simulink model "sudoku"  (R2012b)
settings: Solver=ode45  StartTime=0.0  StopTime=10.0  RelTol=1e-3
libraries: sldvlib x83
(part 4 of 4)

== system sudoku/blocks/block_5 ==
  In1 : Inport
  In2 : Inport  Port=2
  In3 : Inport  Port=3
  In4 : Inport  Port=4
  In5 : Inport  Port=5
  In6 : Inport  Port=6
  In7 : Inport  Port=7
  In8 : Inport  Port=8
  In9 : Inport  Port=9
  Logical Operator : Logic  Inputs=8  AllPortsSameDT=off  OutDataTypeStr=boolean
  Logical Operator1 : Logic  Inputs=7  AllPortsSameDT=off  OutDataTypeStr=boolean
  Logical Operator2 : Logic  Inputs=6  AllPortsSameDT=off  OutDataTypeStr=boolean
  Logical Operator3 : Logic  Inputs=5  AllPortsSameDT=off  OutDataTypeStr=boolean
  Logical Operator4 : Logic  Inputs=4  AllPortsSameDT=off  OutDataTypeStr=boolean
  Logical Operator5 : Logic  Inputs=3  AllPortsSameDT=off  OutDataTypeStr=boolean
  Logical Operator6 : Logic  AllPortsSameDT=off  OutDataTypeStr=boolean
  Logical Operator7 : Logic  Inputs=8  AllPortsSameDT=off  OutDataTypeStr=boolean
  diff{1..36} (36 alike) : RelationalOperator  Operator=~=  OutDataTypeStr=boolean
  Out1 : Outport
  wires:
  In2/1 -> diff1/2, diff15/1, diff14/1, diff13/1, diff12/1, diff11/1, diff10/1, diff9/1
  In1/1 -> diff8/1, diff7/1, diff6/1, diff5/1, diff4/1, diff3/1, diff2/1, diff1/1
  In5/1 -> diff30/1, diff29/1, diff28/1, diff27/1, diff22/2, diff17/2, diff11/2, diff4/2
  In6/1 -> diff33/1, diff32/1, diff31/1, diff27/2, diff23/2, diff18/2, diff12/2, diff5/2
  In7/1 -> diff19/2, diff35/1, diff34/1, diff31/2, diff28/2, diff24/2, diff13/2, diff6/2
  diff1/1 -> Logical Operator/1
  In3/1 -> diff2/2, diff21/1, diff20/1, diff19/1, diff18/1, diff17/1, diff16/1, diff9/2
  In4/1 -> diff26/1, diff25/1, diff24/1, diff23/1, diff22/1, diff16/2, diff10/2, diff3/2
  diff8/1 -> Logical Operator/8
  diff26/1 -> Logical Operator3/5
  diff36/1 -> Logical Operator7/1
  Logical Operator1/1 -> Logical Operator7/7
  diff10/1 -> Logical Operator1/2
  diff18/1 -> Logical Operator2/3
  diff17/1 -> Logical Operator2/2
  diff31/1 -> Logical Operator5/1
  Logical Operator5/1 -> Logical Operator7/3
  diff34/1 -> Logical Operator6/1
  diff16/1 -> Logical Operator2/1
  diff33/1 -> Logical Operator5/3
  diff22/1 -> Logical Operator3/1
  diff35/1 -> Logical Operator6/2
  diff27/1 -> Logical Operator4/1
  Logical Operator/1 -> Logical Operator7/8
  diff25/1 -> Logical Operator3/4
  diff3/1 -> Logical Operator/3
  diff2/1 -> Logical Operator/2
  diff7/1 -> Logical Operator/7
  diff5/1 -> Logical Operator/5
  diff4/1 -> Logical Operator/4
  diff30/1 -> Logical Operator4/4
  Logical Operator7/1 -> Out1/1
  Logical Operator3/1 -> Logical Operator7/5
  Logical Operator6/1 -> Logical Operator7/2
  diff14/1 -> Logical Operator1/6
  Logical Operator2/1 -> Logical Operator7/6
  diff15/1 -> Logical Operator1/7
  diff32/1 -> Logical Operator5/2
  diff21/1 -> Logical Operator2/6
  Logical Operator4/1 -> Logical Operator7/4
  diff19/1 -> Logical Operator2/4
  diff20/1 -> Logical Operator2/5
  diff28/1 -> Logical Operator4/2
  In8/1 -> diff29/2, diff36/1, diff34/2, diff32/2, diff25/2, diff20/2, diff14/2, diff7/2
  diff29/1 -> Logical Operator4/3
  diff6/1 -> Logical Operator/6
  diff9/1 -> Logical Operator1/1
  diff23/1 -> Logical Operator3/2
  diff13/1 -> Logical Operator1/5
  diff24/1 -> Logical Operator3/3
  diff11/1 -> Logical Operator1/3
  diff12/1 -> Logical Operator1/4
  In9/1 -> diff35/2, diff36/2, diff33/2, diff30/2, diff26/2, diff21/2, diff15/2, diff8/2

== system sudoku/blocks/block_6 ==
  In1 : Inport
  In2 : Inport  Port=2
  In3 : Inport  Port=3
  In4 : Inport  Port=4
  In5 : Inport  Port=5
  In6 : Inport  Port=6
  In7 : Inport  Port=7
  In8 : Inport  Port=8
  In9 : Inport  Port=9
  Logical Operator : Logic  Inputs=8  AllPortsSameDT=off  OutDataTypeStr=boolean
  Logical Operator1 : Logic  Inputs=7  AllPortsSameDT=off  OutDataTypeStr=boolean
  Logical Operator2 : Logic  Inputs=6  AllPortsSameDT=off  OutDataTypeStr=boolean
  Logical Operator3 : Logic  Inputs=5  AllPortsSameDT=off  OutDataTypeStr=boolean
  Logical Operator4 : Logic  Inputs=4  AllPortsSameDT=off  OutDataTypeStr=boolean
  Logical Operator5 : Logic  Inputs=3  AllPortsSameDT=off  OutDataTypeStr=boolean
  Logical Operator6 : Logic  AllPortsSameDT=off  OutDataTypeStr=boolean
  Logical Operator7 : Logic  Inputs=8  AllPortsSameDT=off  OutDataTypeStr=boolean
  diff{1..36} (36 alike) : RelationalOperator  Operator=~=  OutDataTypeStr=boolean
  Out1 : Outport
  wires:
  In2/1 -> diff1/2, diff15/1, diff14/1, diff13/1, diff12/1, diff11/1, diff10/1, diff9/1
  In1/1 -> diff8/1, diff7/1, diff6/1, diff5/1, diff4/1, diff3/1, diff2/1, diff1/1
  In5/1 -> diff30/1, diff29/1, diff28/1, diff27/1, diff22/2, diff17/2, diff11/2, diff4/2
  In6/1 -> diff33/1, diff32/1, diff31/1, diff27/2, diff23/2, diff18/2, diff12/2, diff5/2
  In7/1 -> diff19/2, diff35/1, diff34/1, diff31/2, diff28/2, diff24/2, diff13/2, diff6/2
  diff1/1 -> Logical Operator/1
  In3/1 -> diff2/2, diff21/1, diff20/1, diff19/1, diff18/1, diff17/1, diff16/1, diff9/2
  In4/1 -> diff26/1, diff25/1, diff24/1, diff23/1, diff22/1, diff16/2, diff10/2, diff3/2
  diff8/1 -> Logical Operator/8
  diff26/1 -> Logical Operator3/5
  diff36/1 -> Logical Operator7/1
  Logical Operator1/1 -> Logical Operator7/7
  diff10/1 -> Logical Operator1/2
  diff18/1 -> Logical Operator2/3
  diff17/1 -> Logical Operator2/2
  diff31/1 -> Logical Operator5/1
  Logical Operator5/1 -> Logical Operator7/3
  diff34/1 -> Logical Operator6/1
  diff16/1 -> Logical Operator2/1
  diff33/1 -> Logical Operator5/3
  diff22/1 -> Logical Operator3/1
  diff35/1 -> Logical Operator6/2
  diff27/1 -> Logical Operator4/1
  Logical Operator/1 -> Logical Operator7/8
  diff25/1 -> Logical Operator3/4
  diff3/1 -> Logical Operator/3
  diff2/1 -> Logical Operator/2
  diff7/1 -> Logical Operator/7
  diff5/1 -> Logical Operator/5
  diff4/1 -> Logical Operator/4
  diff30/1 -> Logical Operator4/4
  Logical Operator7/1 -> Out1/1
  Logical Operator3/1 -> Logical Operator7/5
  Logical Operator6/1 -> Logical Operator7/2
  diff14/1 -> Logical Operator1/6
  Logical Operator2/1 -> Logical Operator7/6
  diff15/1 -> Logical Operator1/7
  diff32/1 -> Logical Operator5/2
  diff21/1 -> Logical Operator2/6
  Logical Operator4/1 -> Logical Operator7/4
  diff19/1 -> Logical Operator2/4
  diff20/1 -> Logical Operator2/5
  diff28/1 -> Logical Operator4/2
  In8/1 -> diff29/2, diff36/1, diff34/2, diff32/2, diff25/2, diff20/2, diff14/2, diff7/2
  diff29/1 -> Logical Operator4/3
  diff6/1 -> Logical Operator/6
  diff9/1 -> Logical Operator1/1
  diff23/1 -> Logical Operator3/2
  diff13/1 -> Logical Operator1/5
  diff24/1 -> Logical Operator3/3
  diff11/1 -> Logical Operator1/3
  diff12/1 -> Logical Operator1/4
  In9/1 -> diff35/2, diff36/2, diff33/2, diff30/2, diff26/2, diff21/2, diff15/2, diff8/2

== system sudoku/blocks/block_7 ==
  In1 : Inport
  In2 : Inport  Port=2
  In3 : Inport  Port=3
  In4 : Inport  Port=4
  In5 : Inport  Port=5
  In6 : Inport  Port=6
  In7 : Inport  Port=7
  In8 : Inport  Port=8
  In9 : Inport  Port=9
  Logical Operator : Logic  Inputs=8  AllPortsSameDT=off  OutDataTypeStr=boolean
  Logical Operator1 : Logic  Inputs=7  AllPortsSameDT=off  OutDataTypeStr=boolean
  Logical Operator2 : Logic  Inputs=6  AllPortsSameDT=off  OutDataTypeStr=boolean
  Logical Operator3 : Logic  Inputs=5  AllPortsSameDT=off  OutDataTypeStr=boolean
  Logical Operator4 : Logic  Inputs=4  AllPortsSameDT=off  OutDataTypeStr=boolean
  Logical Operator5 : Logic  Inputs=3  AllPortsSameDT=off  OutDataTypeStr=boolean
  Logical Operator6 : Logic  AllPortsSameDT=off  OutDataTypeStr=boolean
  Logical Operator7 : Logic  Inputs=8  AllPortsSameDT=off  OutDataTypeStr=boolean
  diff{1..36} (36 alike) : RelationalOperator  Operator=~=  OutDataTypeStr=boolean
  Out1 : Outport
  wires:
  In2/1 -> diff1/2, diff15/1, diff14/1, diff13/1, diff12/1, diff11/1, diff10/1, diff9/1
  In1/1 -> diff8/1, diff7/1, diff6/1, diff5/1, diff4/1, diff3/1, diff2/1, diff1/1
  In5/1 -> diff30/1, diff29/1, diff28/1, diff27/1, diff22/2, diff17/2, diff11/2, diff4/2
  In6/1 -> diff33/1, diff32/1, diff31/1, diff27/2, diff23/2, diff18/2, diff12/2, diff5/2
  In7/1 -> diff19/2, diff35/1, diff34/1, diff31/2, diff28/2, diff24/2, diff13/2, diff6/2
  diff1/1 -> Logical Operator/1
  In3/1 -> diff2/2, diff21/1, diff20/1, diff19/1, diff18/1, diff17/1, diff16/1, diff9/2
  In4/1 -> diff26/1, diff25/1, diff24/1, diff23/1, diff22/1, diff16/2, diff10/2, diff3/2
  diff8/1 -> Logical Operator/8
  diff26/1 -> Logical Operator3/5
  diff36/1 -> Logical Operator7/1
  Logical Operator1/1 -> Logical Operator7/7
  diff10/1 -> Logical Operator1/2
  diff18/1 -> Logical Operator2/3
  diff17/1 -> Logical Operator2/2
  diff31/1 -> Logical Operator5/1
  Logical Operator5/1 -> Logical Operator7/3
  diff34/1 -> Logical Operator6/1
  diff16/1 -> Logical Operator2/1
  diff33/1 -> Logical Operator5/3
  diff22/1 -> Logical Operator3/1
  diff35/1 -> Logical Operator6/2
  diff27/1 -> Logical Operator4/1
  Logical Operator/1 -> Logical Operator7/8
  diff25/1 -> Logical Operator3/4
  diff3/1 -> Logical Operator/3
  diff2/1 -> Logical Operator/2
  diff7/1 -> Logical Operator/7
  diff5/1 -> Logical Operator/5
  diff4/1 -> Logical Operator/4
  diff30/1 -> Logical Operator4/4
  Logical Operator7/1 -> Out1/1
  Logical Operator3/1 -> Logical Operator7/5
  Logical Operator6/1 -> Logical Operator7/2
  diff14/1 -> Logical Operator1/6
  Logical Operator2/1 -> Logical Operator7/6
  diff15/1 -> Logical Operator1/7
  diff32/1 -> Logical Operator5/2
  diff21/1 -> Logical Operator2/6
  Logical Operator4/1 -> Logical Operator7/4
  diff19/1 -> Logical Operator2/4
  diff20/1 -> Logical Operator2/5
  diff28/1 -> Logical Operator4/2
  In8/1 -> diff29/2, diff36/1, diff34/2, diff32/2, diff25/2, diff20/2, diff14/2, diff7/2
  diff29/1 -> Logical Operator4/3
  diff6/1 -> Logical Operator/6
  diff9/1 -> Logical Operator1/1
  diff23/1 -> Logical Operator3/2
  diff13/1 -> Logical Operator1/5
  diff24/1 -> Logical Operator3/3
  diff11/1 -> Logical Operator1/3
  diff12/1 -> Logical Operator1/4
  In9/1 -> diff35/2, diff36/2, diff33/2, diff30/2, diff26/2, diff21/2, diff15/2, diff8/2

== system sudoku/blocks/block_8 ==
  In1 : Inport
  In2 : Inport  Port=2
  In3 : Inport  Port=3
  In4 : Inport  Port=4
  In5 : Inport  Port=5
  In6 : Inport  Port=6
  In7 : Inport  Port=7
  In8 : Inport  Port=8
  In9 : Inport  Port=9
  Logical Operator : Logic  Inputs=8  AllPortsSameDT=off  OutDataTypeStr=boolean
  Logical Operator1 : Logic  Inputs=7  AllPortsSameDT=off  OutDataTypeStr=boolean
  Logical Operator2 : Logic  Inputs=6  AllPortsSameDT=off  OutDataTypeStr=boolean
  Logical Operator3 : Logic  Inputs=5  AllPortsSameDT=off  OutDataTypeStr=boolean
  Logical Operator4 : Logic  Inputs=4  AllPortsSameDT=off  OutDataTypeStr=boolean
  Logical Operator5 : Logic  Inputs=3  AllPortsSameDT=off  OutDataTypeStr=boolean
  Logical Operator6 : Logic  AllPortsSameDT=off  OutDataTypeStr=boolean
  Logical Operator7 : Logic  Inputs=8  AllPortsSameDT=off  OutDataTypeStr=boolean
  diff{1..36} (36 alike) : RelationalOperator  Operator=~=  OutDataTypeStr=boolean
  Out1 : Outport
  wires:
  In2/1 -> diff1/2, diff15/1, diff14/1, diff13/1, diff12/1, diff11/1, diff10/1, diff9/1
  In1/1 -> diff8/1, diff7/1, diff6/1, diff5/1, diff4/1, diff3/1, diff2/1, diff1/1
  In5/1 -> diff30/1, diff29/1, diff28/1, diff27/1, diff22/2, diff17/2, diff11/2, diff4/2
  In6/1 -> diff33/1, diff32/1, diff31/1, diff27/2, diff23/2, diff18/2, diff12/2, diff5/2
  In7/1 -> diff19/2, diff35/1, diff34/1, diff31/2, diff28/2, diff24/2, diff13/2, diff6/2
  diff1/1 -> Logical Operator/1
  In3/1 -> diff2/2, diff21/1, diff20/1, diff19/1, diff18/1, diff17/1, diff16/1, diff9/2
  In4/1 -> diff26/1, diff25/1, diff24/1, diff23/1, diff22/1, diff16/2, diff10/2, diff3/2
  diff8/1 -> Logical Operator/8
  diff26/1 -> Logical Operator3/5
  diff36/1 -> Logical Operator7/1
  Logical Operator1/1 -> Logical Operator7/7
  diff10/1 -> Logical Operator1/2
  diff18/1 -> Logical Operator2/3
  diff17/1 -> Logical Operator2/2
  diff31/1 -> Logical Operator5/1
  Logical Operator5/1 -> Logical Operator7/3
  diff34/1 -> Logical Operator6/1
  diff16/1 -> Logical Operator2/1
  diff33/1 -> Logical Operator5/3
  diff22/1 -> Logical Operator3/1
  diff35/1 -> Logical Operator6/2
  diff27/1 -> Logical Operator4/1
  Logical Operator/1 -> Logical Operator7/8
  diff25/1 -> Logical Operator3/4
  diff3/1 -> Logical Operator/3
  diff2/1 -> Logical Operator/2
  diff7/1 -> Logical Operator/7
  diff5/1 -> Logical Operator/5
  diff4/1 -> Logical Operator/4
  diff30/1 -> Logical Operator4/4
  Logical Operator7/1 -> Out1/1
  Logical Operator3/1 -> Logical Operator7/5
  Logical Operator6/1 -> Logical Operator7/2
  diff14/1 -> Logical Operator1/6
  Logical Operator2/1 -> Logical Operator7/6
  diff15/1 -> Logical Operator1/7
  diff32/1 -> Logical Operator5/2
  diff21/1 -> Logical Operator2/6
  Logical Operator4/1 -> Logical Operator7/4
  diff19/1 -> Logical Operator2/4
  diff20/1 -> Logical Operator2/5
  diff28/1 -> Logical Operator4/2
  In8/1 -> diff29/2, diff36/1, diff34/2, diff32/2, diff25/2, diff20/2, diff14/2, diff7/2
  diff29/1 -> Logical Operator4/3
  diff6/1 -> Logical Operator/6
  diff9/1 -> Logical Operator1/1
  diff23/1 -> Logical Operator3/2
  diff13/1 -> Logical Operator1/5
  diff24/1 -> Logical Operator3/3
  diff11/1 -> Logical Operator1/3
  diff12/1 -> Logical Operator1/4
  In9/1 -> diff35/2, diff36/2, diff33/2, diff30/2, diff26/2, diff21/2, diff15/2, diff8/2

== system sudoku/blocks/block_9 ==
  In1 : Inport
  In2 : Inport  Port=2
  In3 : Inport  Port=3
  In4 : Inport  Port=4
  In5 : Inport  Port=5
  In6 : Inport  Port=6
  In7 : Inport  Port=7
  In8 : Inport  Port=8
  In9 : Inport  Port=9
  Logical Operator : Logic  Inputs=8  AllPortsSameDT=off  OutDataTypeStr=boolean
  Logical Operator1 : Logic  Inputs=7  AllPortsSameDT=off  OutDataTypeStr=boolean
  Logical Operator2 : Logic  Inputs=6  AllPortsSameDT=off  OutDataTypeStr=boolean
  Logical Operator3 : Logic  Inputs=5  AllPortsSameDT=off  OutDataTypeStr=boolean
  Logical Operator4 : Logic  Inputs=4  AllPortsSameDT=off  OutDataTypeStr=boolean
  Logical Operator5 : Logic  Inputs=3  AllPortsSameDT=off  OutDataTypeStr=boolean
  Logical Operator6 : Logic  AllPortsSameDT=off  OutDataTypeStr=boolean
  Logical Operator7 : Logic  Inputs=8  AllPortsSameDT=off  OutDataTypeStr=boolean
  diff{1..36} (36 alike) : RelationalOperator  Operator=~=  OutDataTypeStr=boolean
  Out1 : Outport
  wires:
  In2/1 -> diff1/2, diff15/1, diff14/1, diff13/1, diff12/1, diff11/1, diff10/1, diff9/1
  In1/1 -> diff8/1, diff7/1, diff6/1, diff5/1, diff4/1, diff3/1, diff2/1, diff1/1
  In5/1 -> diff30/1, diff29/1, diff28/1, diff27/1, diff22/2, diff17/2, diff11/2, diff4/2
  In6/1 -> diff33/1, diff32/1, diff31/1, diff27/2, diff23/2, diff18/2, diff12/2, diff5/2
  In7/1 -> diff19/2, diff35/1, diff34/1, diff31/2, diff28/2, diff24/2, diff13/2, diff6/2
  diff1/1 -> Logical Operator/1
  In3/1 -> diff2/2, diff21/1, diff20/1, diff19/1, diff18/1, diff17/1, diff16/1, diff9/2
  In4/1 -> diff26/1, diff25/1, diff24/1, diff23/1, diff22/1, diff16/2, diff10/2, diff3/2
  diff8/1 -> Logical Operator/8
  diff26/1 -> Logical Operator3/5
  diff36/1 -> Logical Operator7/1
  Logical Operator1/1 -> Logical Operator7/7
  diff10/1 -> Logical Operator1/2
  diff18/1 -> Logical Operator2/3
  diff17/1 -> Logical Operator2/2
  diff31/1 -> Logical Operator5/1
  Logical Operator5/1 -> Logical Operator7/3
  diff34/1 -> Logical Operator6/1
  diff16/1 -> Logical Operator2/1
  diff33/1 -> Logical Operator5/3
  diff22/1 -> Logical Operator3/1
  diff35/1 -> Logical Operator6/2
  diff27/1 -> Logical Operator4/1
  Logical Operator/1 -> Logical Operator7/8
  diff25/1 -> Logical Operator3/4
  diff3/1 -> Logical Operator/3
  diff2/1 -> Logical Operator/2
  diff7/1 -> Logical Operator/7
  diff5/1 -> Logical Operator/5
  diff4/1 -> Logical Operator/4
  diff30/1 -> Logical Operator4/4
  Logical Operator7/1 -> Out1/1
  Logical Operator3/1 -> Logical Operator7/5
  Logical Operator6/1 -> Logical Operator7/2
  diff14/1 -> Logical Operator1/6
  Logical Operator2/1 -> Logical Operator7/6
  diff15/1 -> Logical Operator1/7
  diff32/1 -> Logical Operator5/2
  diff21/1 -> Logical Operator2/6
  Logical Operator4/1 -> Logical Operator7/4
  diff19/1 -> Logical Operator2/4
  diff20/1 -> Logical Operator2/5
  diff28/1 -> Logical Operator4/2
  In8/1 -> diff29/2, diff36/1, diff34/2, diff32/2, diff25/2, diff20/2, diff14/2, diff7/2
  diff29/1 -> Logical Operator4/3
  diff6/1 -> Logical Operator/6
  diff9/1 -> Logical Operator1/1
  diff23/1 -> Logical Operator3/2
  diff13/1 -> Logical Operator1/5
  diff24/1 -> Logical Operator3/3
  diff11/1 -> Logical Operator1/3
  diff12/1 -> Logical Operator1/4
  In9/1 -> diff35/2, diff36/2, diff33/2, diff30/2, diff26/2, diff21/2, diff15/2, diff8/2

== system sudoku/columns/col_1 ==
  In1 : Inport
  In2 : Inport  Port=2
  In3 : Inport  Port=3
  In4 : Inport  Port=4
  In5 : Inport  Port=5
  In6 : Inport  Port=6
  In7 : Inport  Port=7
  In8 : Inport  Port=8
  In9 : Inport  Port=9
  Logical Operator : Logic  Inputs=8  AllPortsSameDT=off  OutDataTypeStr=boolean
  Logical Operator1 : Logic  Inputs=7  AllPortsSameDT=off  OutDataTypeStr=boolean
  Logical Operator2 : Logic  Inputs=6  AllPortsSameDT=off  OutDataTypeStr=boolean
  Logical Operator3 : Logic  Inputs=5  AllPortsSameDT=off  OutDataTypeStr=boolean
  Logical Operator4 : Logic  Inputs=4  AllPortsSameDT=off  OutDataTypeStr=boolean
  Logical Operator5 : Logic  Inputs=3  AllPortsSameDT=off  OutDataTypeStr=boolean
  Logical Operator6 : Logic  AllPortsSameDT=off  OutDataTypeStr=boolean
  Logical Operator7 : Logic  Inputs=8  AllPortsSameDT=off  OutDataTypeStr=boolean
  diff{1..36} (36 alike) : RelationalOperator  Operator=~=  OutDataTypeStr=boolean
  Out1 : Outport
  wires:
  In2/1 -> diff1/2, diff15/1, diff14/1, diff13/1, diff12/1, diff11/1, diff10/1, diff9/1
  In1/1 -> diff8/1, diff7/1, diff6/1, diff5/1, diff4/1, diff3/1, diff2/1, diff1/1
  In5/1 -> diff30/1, diff29/1, diff28/1, diff27/1, diff22/2, diff17/2, diff11/2, diff4/2
  In6/1 -> diff33/1, diff32/1, diff31/1, diff27/2, diff23/2, diff18/2, diff12/2, diff5/2
  In7/1 -> diff19/2, diff35/1, diff34/1, diff31/2, diff28/2, diff24/2, diff13/2, diff6/2
  diff1/1 -> Logical Operator/1
  In3/1 -> diff2/2, diff21/1, diff20/1, diff19/1, diff18/1, diff17/1, diff16/1, diff9/2
  In4/1 -> diff26/1, diff25/1, diff24/1, diff23/1, diff22/1, diff16/2, diff10/2, diff3/2
  diff8/1 -> Logical Operator/8
  diff26/1 -> Logical Operator3/5
  diff36/1 -> Logical Operator7/1
  Logical Operator1/1 -> Logical Operator7/7
  diff10/1 -> Logical Operator1/2
  diff18/1 -> Logical Operator2/3
  diff17/1 -> Logical Operator2/2
  diff31/1 -> Logical Operator5/1
  Logical Operator5/1 -> Logical Operator7/3
  diff34/1 -> Logical Operator6/1
  diff16/1 -> Logical Operator2/1
  diff33/1 -> Logical Operator5/3
  diff22/1 -> Logical Operator3/1
  diff35/1 -> Logical Operator6/2
  diff27/1 -> Logical Operator4/1
  Logical Operator/1 -> Logical Operator7/8
  diff25/1 -> Logical Operator3/4
  diff3/1 -> Logical Operator/3
  diff2/1 -> Logical Operator/2
  diff7/1 -> Logical Operator/7
  diff5/1 -> Logical Operator/5
  diff4/1 -> Logical Operator/4
  diff30/1 -> Logical Operator4/4
  Logical Operator7/1 -> Out1/1
  Logical Operator3/1 -> Logical Operator7/5
  Logical Operator6/1 -> Logical Operator7/2
  diff14/1 -> Logical Operator1/6
  Logical Operator2/1 -> Logical Operator7/6
  diff15/1 -> Logical Operator1/7
  diff32/1 -> Logical Operator5/2
  diff21/1 -> Logical Operator2/6
  Logical Operator4/1 -> Logical Operator7/4
  diff19/1 -> Logical Operator2/4
  diff20/1 -> Logical Operator2/5
  diff28/1 -> Logical Operator4/2
  In8/1 -> diff29/2, diff36/1, diff34/2, diff32/2, diff25/2, diff20/2, diff14/2, diff7/2
  diff29/1 -> Logical Operator4/3
  diff6/1 -> Logical Operator/6
  diff9/1 -> Logical Operator1/1
  diff23/1 -> Logical Operator3/2
  diff13/1 -> Logical Operator1/5
  diff24/1 -> Logical Operator3/3
  diff11/1 -> Logical Operator1/3
  diff12/1 -> Logical Operator1/4
  In9/1 -> diff35/2, diff36/2, diff33/2, diff30/2, diff26/2, diff21/2, diff15/2, diff8/2

== system sudoku/columns/col_2 ==
  In1 : Inport
  In2 : Inport  Port=2
  In3 : Inport  Port=3
  In4 : Inport  Port=4
  In5 : Inport  Port=5
  In6 : Inport  Port=6
  In7 : Inport  Port=7
  In8 : Inport  Port=8
  In9 : Inport  Port=9
  Logical Operator : Logic  Inputs=8  AllPortsSameDT=off  OutDataTypeStr=boolean
  Logical Operator1 : Logic  Inputs=7  AllPortsSameDT=off  OutDataTypeStr=boolean
  Logical Operator2 : Logic  Inputs=6  AllPortsSameDT=off  OutDataTypeStr=boolean
  Logical Operator3 : Logic  Inputs=5  AllPortsSameDT=off  OutDataTypeStr=boolean
  Logical Operator4 : Logic  Inputs=4  AllPortsSameDT=off  OutDataTypeStr=boolean
  Logical Operator5 : Logic  Inputs=3  AllPortsSameDT=off  OutDataTypeStr=boolean
  Logical Operator6 : Logic  AllPortsSameDT=off  OutDataTypeStr=boolean
  Logical Operator7 : Logic  Inputs=8  AllPortsSameDT=off  OutDataTypeStr=boolean
  diff{1..36} (36 alike) : RelationalOperator  Operator=~=  OutDataTypeStr=boolean
  Out1 : Outport
  wires:
  In2/1 -> diff1/2, diff15/1, diff14/1, diff13/1, diff12/1, diff11/1, diff10/1, diff9/1
  In1/1 -> diff8/1, diff7/1, diff6/1, diff5/1, diff4/1, diff3/1, diff2/1, diff1/1
  In5/1 -> diff30/1, diff29/1, diff28/1, diff27/1, diff22/2, diff17/2, diff11/2, diff4/2
  In6/1 -> diff33/1, diff32/1, diff31/1, diff27/2, diff23/2, diff18/2, diff12/2, diff5/2
  In7/1 -> diff19/2, diff35/1, diff34/1, diff31/2, diff28/2, diff24/2, diff13/2, diff6/2
  diff1/1 -> Logical Operator/1
  In3/1 -> diff2/2, diff21/1, diff20/1, diff19/1, diff18/1, diff17/1, diff16/1, diff9/2
  In4/1 -> diff26/1, diff25/1, diff24/1, diff23/1, diff22/1, diff16/2, diff10/2, diff3/2
  diff8/1 -> Logical Operator/8
  diff26/1 -> Logical Operator3/5
  diff36/1 -> Logical Operator7/1
  Logical Operator1/1 -> Logical Operator7/7
  diff10/1 -> Logical Operator1/2
  diff18/1 -> Logical Operator2/3
  diff17/1 -> Logical Operator2/2
  diff31/1 -> Logical Operator5/1
  Logical Operator5/1 -> Logical Operator7/3
  diff34/1 -> Logical Operator6/1
  diff16/1 -> Logical Operator2/1
  diff33/1 -> Logical Operator5/3
  diff22/1 -> Logical Operator3/1
  diff35/1 -> Logical Operator6/2
  diff27/1 -> Logical Operator4/1
  Logical Operator/1 -> Logical Operator7/8
  diff25/1 -> Logical Operator3/4
  diff3/1 -> Logical Operator/3
  diff2/1 -> Logical Operator/2
  diff7/1 -> Logical Operator/7
  diff5/1 -> Logical Operator/5
  diff4/1 -> Logical Operator/4
  diff30/1 -> Logical Operator4/4
  Logical Operator7/1 -> Out1/1
  Logical Operator3/1 -> Logical Operator7/5
  Logical Operator6/1 -> Logical Operator7/2
  diff14/1 -> Logical Operator1/6
  Logical Operator2/1 -> Logical Operator7/6
  diff15/1 -> Logical Operator1/7
  diff32/1 -> Logical Operator5/2
  diff21/1 -> Logical Operator2/6
  Logical Operator4/1 -> Logical Operator7/4
  diff19/1 -> Logical Operator2/4
  diff20/1 -> Logical Operator2/5
  diff28/1 -> Logical Operator4/2
  In8/1 -> diff29/2, diff36/1, diff34/2, diff32/2, diff25/2, diff20/2, diff14/2, diff7/2
  diff29/1 -> Logical Operator4/3
  diff6/1 -> Logical Operator/6
  diff9/1 -> Logical Operator1/1
  diff23/1 -> Logical Operator3/2
  diff13/1 -> Logical Operator1/5
  diff24/1 -> Logical Operator3/3
  diff11/1 -> Logical Operator1/3
  diff12/1 -> Logical Operator1/4
  In9/1 -> diff35/2, diff36/2, diff33/2, diff30/2, diff26/2, diff21/2, diff15/2, diff8/2

== system sudoku/columns/col_3 ==
  In1 : Inport
  In2 : Inport  Port=2
  In3 : Inport  Port=3
  In4 : Inport  Port=4
  In5 : Inport  Port=5
  In6 : Inport  Port=6
  In7 : Inport  Port=7
  In8 : Inport  Port=8
  In9 : Inport  Port=9
  Logical Operator : Logic  Inputs=8  AllPortsSameDT=off  OutDataTypeStr=boolean
  Logical Operator1 : Logic  Inputs=7  AllPortsSameDT=off  OutDataTypeStr=boolean
  Logical Operator2 : Logic  Inputs=6  AllPortsSameDT=off  OutDataTypeStr=boolean
  Logical Operator3 : Logic  Inputs=5  AllPortsSameDT=off  OutDataTypeStr=boolean
  Logical Operator4 : Logic  Inputs=4  AllPortsSameDT=off  OutDataTypeStr=boolean
  Logical Operator5 : Logic  Inputs=3  AllPortsSameDT=off  OutDataTypeStr=boolean
  Logical Operator6 : Logic  AllPortsSameDT=off  OutDataTypeStr=boolean
  Logical Operator7 : Logic  Inputs=8  AllPortsSameDT=off  OutDataTypeStr=boolean
  diff{1..36} (36 alike) : RelationalOperator  Operator=~=  OutDataTypeStr=boolean
  Out1 : Outport
  wires:
  In2/1 -> diff1/2, diff15/1, diff14/1, diff13/1, diff12/1, diff11/1, diff10/1, diff9/1
  In1/1 -> diff8/1, diff7/1, diff6/1, diff5/1, diff4/1, diff3/1, diff2/1, diff1/1
  In5/1 -> diff30/1, diff29/1, diff28/1, diff27/1, diff22/2, diff17/2, diff11/2, diff4/2
  In6/1 -> diff33/1, diff32/1, diff31/1, diff27/2, diff23/2, diff18/2, diff12/2, diff5/2
  In7/1 -> diff19/2, diff35/1, diff34/1, diff31/2, diff28/2, diff24/2, diff13/2, diff6/2
  diff1/1 -> Logical Operator/1
  In3/1 -> diff2/2, diff21/1, diff20/1, diff19/1, diff18/1, diff17/1, diff16/1, diff9/2
  In4/1 -> diff26/1, diff25/1, diff24/1, diff23/1, diff22/1, diff16/2, diff10/2, diff3/2
  diff8/1 -> Logical Operator/8
  diff26/1 -> Logical Operator3/5
  diff36/1 -> Logical Operator7/1
  Logical Operator1/1 -> Logical Operator7/7
  diff10/1 -> Logical Operator1/2
  diff18/1 -> Logical Operator2/3
  diff17/1 -> Logical Operator2/2
  diff31/1 -> Logical Operator5/1
  Logical Operator5/1 -> Logical Operator7/3
  diff34/1 -> Logical Operator6/1
  diff16/1 -> Logical Operator2/1
  diff33/1 -> Logical Operator5/3
  diff22/1 -> Logical Operator3/1
  diff35/1 -> Logical Operator6/2
  diff27/1 -> Logical Operator4/1
  Logical Operator/1 -> Logical Operator7/8
  diff25/1 -> Logical Operator3/4
  diff3/1 -> Logical Operator/3
  diff2/1 -> Logical Operator/2
  diff7/1 -> Logical Operator/7
  diff5/1 -> Logical Operator/5
  diff4/1 -> Logical Operator/4
  diff30/1 -> Logical Operator4/4
  Logical Operator7/1 -> Out1/1
  Logical Operator3/1 -> Logical Operator7/5
  Logical Operator6/1 -> Logical Operator7/2
  diff14/1 -> Logical Operator1/6
  Logical Operator2/1 -> Logical Operator7/6
  diff15/1 -> Logical Operator1/7
  diff32/1 -> Logical Operator5/2
  diff21/1 -> Logical Operator2/6
  Logical Operator4/1 -> Logical Operator7/4
  diff19/1 -> Logical Operator2/4
  diff20/1 -> Logical Operator2/5
  diff28/1 -> Logical Operator4/2
  In8/1 -> diff29/2, diff36/1, diff34/2, diff32/2, diff25/2, diff20/2, diff14/2, diff7/2
  diff29/1 -> Logical Operator4/3
  diff6/1 -> Logical Operator/6
  diff9/1 -> Logical Operator1/1
  diff23/1 -> Logical Operator3/2
  diff13/1 -> Logical Operator1/5
  diff24/1 -> Logical Operator3/3
  diff11/1 -> Logical Operator1/3
  diff12/1 -> Logical Operator1/4
  In9/1 -> diff35/2, diff36/2, diff33/2, diff30/2, diff26/2, diff21/2, diff15/2, diff8/2

== system sudoku/columns/col_4 ==
  In1 : Inport
  In2 : Inport  Port=2
  In3 : Inport  Port=3
  In4 : Inport  Port=4
  In5 : Inport  Port=5
  In6 : Inport  Port=6
  In7 : Inport  Port=7
  In8 : Inport  Port=8
  In9 : Inport  Port=9
  Logical Operator : Logic  Inputs=8  AllPortsSameDT=off  OutDataTypeStr=boolean
  Logical Operator1 : Logic  Inputs=7  AllPortsSameDT=off  OutDataTypeStr=boolean
  Logical Operator2 : Logic  Inputs=6  AllPortsSameDT=off  OutDataTypeStr=boolean
  Logical Operator3 : Logic  Inputs=5  AllPortsSameDT=off  OutDataTypeStr=boolean
  Logical Operator4 : Logic  Inputs=4  AllPortsSameDT=off  OutDataTypeStr=boolean
  Logical Operator5 : Logic  Inputs=3  AllPortsSameDT=off  OutDataTypeStr=boolean
  Logical Operator6 : Logic  AllPortsSameDT=off  OutDataTypeStr=boolean
  Logical Operator7 : Logic  Inputs=8  AllPortsSameDT=off  OutDataTypeStr=boolean
  diff{1..36} (36 alike) : RelationalOperator  Operator=~=  OutDataTypeStr=boolean
  Out1 : Outport
  wires:
  In2/1 -> diff1/2, diff15/1, diff14/1, diff13/1, diff12/1, diff11/1, diff10/1, diff9/1
  In1/1 -> diff8/1, diff7/1, diff6/1, diff5/1, diff4/1, diff3/1, diff2/1, diff1/1
  In5/1 -> diff30/1, diff29/1, diff28/1, diff27/1, diff22/2, diff17/2, diff11/2, diff4/2
  In6/1 -> diff33/1, diff32/1, diff31/1, diff27/2, diff23/2, diff18/2, diff12/2, diff5/2
  In7/1 -> diff19/2, diff35/1, diff34/1, diff31/2, diff28/2, diff24/2, diff13/2, diff6/2
  diff1/1 -> Logical Operator/1
  In3/1 -> diff2/2, diff21/1, diff20/1, diff19/1, diff18/1, diff17/1, diff16/1, diff9/2
  In4/1 -> diff26/1, diff25/1, diff24/1, diff23/1, diff22/1, diff16/2, diff10/2, diff3/2
  diff8/1 -> Logical Operator/8
  diff26/1 -> Logical Operator3/5
  diff36/1 -> Logical Operator7/1
  Logical Operator1/1 -> Logical Operator7/7
  diff10/1 -> Logical Operator1/2
  diff18/1 -> Logical Operator2/3
  diff17/1 -> Logical Operator2/2
  diff31/1 -> Logical Operator5/1
  Logical Operator5/1 -> Logical Operator7/3
  diff34/1 -> Logical Operator6/1
  diff16/1 -> Logical Operator2/1
  diff33/1 -> Logical Operator5/3
  diff22/1 -> Logical Operator3/1
  diff35/1 -> Logical Operator6/2
  diff27/1 -> Logical Operator4/1
  Logical Operator/1 -> Logical Operator7/8
  diff25/1 -> Logical Operator3/4
  diff3/1 -> Logical Operator/3
  diff2/1 -> Logical Operator/2
  diff7/1 -> Logical Operator/7
  diff5/1 -> Logical Operator/5
  diff4/1 -> Logical Operator/4
  diff30/1 -> Logical Operator4/4
  Logical Operator7/1 -> Out1/1
  Logical Operator3/1 -> Logical Operator7/5
  Logical Operator6/1 -> Logical Operator7/2
  diff14/1 -> Logical Operator1/6
  Logical Operator2/1 -> Logical Operator7/6
  diff15/1 -> Logical Operator1/7
  diff32/1 -> Logical Operator5/2
  diff21/1 -> Logical Operator2/6
  Logical Operator4/1 -> Logical Operator7/4
  diff19/1 -> Logical Operator2/4
  diff20/1 -> Logical Operator2/5
  diff28/1 -> Logical Operator4/2
  In8/1 -> diff29/2, diff36/1, diff34/2, diff32/2, diff25/2, diff20/2, diff14/2, diff7/2
  diff29/1 -> Logical Operator4/3
  diff6/1 -> Logical Operator/6
  diff9/1 -> Logical Operator1/1
  diff23/1 -> Logical Operator3/2
  diff13/1 -> Logical Operator1/5
  diff24/1 -> Logical Operator3/3
  diff11/1 -> Logical Operator1/3
  diff12/1 -> Logical Operator1/4
  In9/1 -> diff35/2, diff36/2, diff33/2, diff30/2, diff26/2, diff21/2, diff15/2, diff8/2

== system sudoku/columns/col_5 ==
  In1 : Inport
  In2 : Inport  Port=2
  In3 : Inport  Port=3
  In4 : Inport  Port=4
  In5 : Inport  Port=5
  In6 : Inport  Port=6
  In7 : Inport  Port=7
  In8 : Inport  Port=8
  In9 : Inport  Port=9
  Logical Operator : Logic  Inputs=8  AllPortsSameDT=off  OutDataTypeStr=boolean
  Logical Operator1 : Logic  Inputs=7  AllPortsSameDT=off  OutDataTypeStr=boolean
  Logical Operator2 : Logic  Inputs=6  AllPortsSameDT=off  OutDataTypeStr=boolean
  Logical Operator3 : Logic  Inputs=5  AllPortsSameDT=off  OutDataTypeStr=boolean
  Logical Operator4 : Logic  Inputs=4  AllPortsSameDT=off  OutDataTypeStr=boolean
  Logical Operator5 : Logic  Inputs=3  AllPortsSameDT=off  OutDataTypeStr=boolean
  Logical Operator6 : Logic  AllPortsSameDT=off  OutDataTypeStr=boolean
  Logical Operator7 : Logic  Inputs=8  AllPortsSameDT=off  OutDataTypeStr=boolean
  diff{1..36} (36 alike) : RelationalOperator  Operator=~=  OutDataTypeStr=boolean
  Out1 : Outport
  wires:
  In2/1 -> diff1/2, diff15/1, diff14/1, diff13/1, diff12/1, diff11/1, diff10/1, diff9/1
  In1/1 -> diff8/1, diff7/1, diff6/1, diff5/1, diff4/1, diff3/1, diff2/1, diff1/1
  In5/1 -> diff30/1, diff29/1, diff28/1, diff27/1, diff22/2, diff17/2, diff11/2, diff4/2
  In6/1 -> diff33/1, diff32/1, diff31/1, diff27/2, diff23/2, diff18/2, diff12/2, diff5/2
  In7/1 -> diff19/2, diff35/1, diff34/1, diff31/2, diff28/2, diff24/2, diff13/2, diff6/2
  diff1/1 -> Logical Operator/1
  In3/1 -> diff2/2, diff21/1, diff20/1, diff19/1, diff18/1, diff17/1, diff16/1, diff9/2
  In4/1 -> diff26/1, diff25/1, diff24/1, diff23/1, diff22/1, diff16/2, diff10/2, diff3/2
  diff8/1 -> Logical Operator/8
  diff26/1 -> Logical Operator3/5
  diff36/1 -> Logical Operator7/1
  Logical Operator1/1 -> Logical Operator7/7
  diff10/1 -> Logical Operator1/2
  diff18/1 -> Logical Operator2/3
  diff17/1 -> Logical Operator2/2
  diff31/1 -> Logical Operator5/1
  Logical Operator5/1 -> Logical Operator7/3
  diff34/1 -> Logical Operator6/1
  diff16/1 -> Logical Operator2/1
  diff33/1 -> Logical Operator5/3
  diff22/1 -> Logical Operator3/1
  diff35/1 -> Logical Operator6/2
  diff27/1 -> Logical Operator4/1
  Logical Operator/1 -> Logical Operator7/8
  diff25/1 -> Logical Operator3/4
  diff3/1 -> Logical Operator/3
  diff2/1 -> Logical Operator/2
  diff7/1 -> Logical Operator/7
  diff5/1 -> Logical Operator/5
  diff4/1 -> Logical Operator/4
  diff30/1 -> Logical Operator4/4
  Logical Operator7/1 -> Out1/1
  Logical Operator3/1 -> Logical Operator7/5
  Logical Operator6/1 -> Logical Operator7/2
  diff14/1 -> Logical Operator1/6
  Logical Operator2/1 -> Logical Operator7/6
  diff15/1 -> Logical Operator1/7
  diff32/1 -> Logical Operator5/2
  diff21/1 -> Logical Operator2/6
  Logical Operator4/1 -> Logical Operator7/4
  diff19/1 -> Logical Operator2/4
  diff20/1 -> Logical Operator2/5
  diff28/1 -> Logical Operator4/2
  In8/1 -> diff29/2, diff36/1, diff34/2, diff32/2, diff25/2, diff20/2, diff14/2, diff7/2
  diff29/1 -> Logical Operator4/3
  diff6/1 -> Logical Operator/6
  diff9/1 -> Logical Operator1/1
  diff23/1 -> Logical Operator3/2
  diff13/1 -> Logical Operator1/5
  diff24/1 -> Logical Operator3/3
  diff11/1 -> Logical Operator1/3
  diff12/1 -> Logical Operator1/4
  In9/1 -> diff35/2, diff36/2, diff33/2, diff30/2, diff26/2, diff21/2, diff15/2, diff8/2

== system sudoku/columns/col_6 ==
  In1 : Inport
  In2 : Inport  Port=2
  In3 : Inport  Port=3
  In4 : Inport  Port=4
  In5 : Inport  Port=5
  In6 : Inport  Port=6
  In7 : Inport  Port=7
  In8 : Inport  Port=8
  In9 : Inport  Port=9
  Logical Operator : Logic  Inputs=8  AllPortsSameDT=off  OutDataTypeStr=boolean
  Logical Operator1 : Logic  Inputs=7  AllPortsSameDT=off  OutDataTypeStr=boolean
  Logical Operator2 : Logic  Inputs=6  AllPortsSameDT=off  OutDataTypeStr=boolean
  Logical Operator3 : Logic  Inputs=5  AllPortsSameDT=off  OutDataTypeStr=boolean
  Logical Operator4 : Logic  Inputs=4  AllPortsSameDT=off  OutDataTypeStr=boolean
  Logical Operator5 : Logic  Inputs=3  AllPortsSameDT=off  OutDataTypeStr=boolean
  Logical Operator6 : Logic  AllPortsSameDT=off  OutDataTypeStr=boolean
  Logical Operator7 : Logic  Inputs=8  AllPortsSameDT=off  OutDataTypeStr=boolean
  diff{1..36} (36 alike) : RelationalOperator  Operator=~=  OutDataTypeStr=boolean
  Out1 : Outport
  wires:
  In2/1 -> diff1/2, diff15/1, diff14/1, diff13/1, diff12/1, diff11/1, diff10/1, diff9/1
  In1/1 -> diff8/1, diff7/1, diff6/1, diff5/1, diff4/1, diff3/1, diff2/1, diff1/1
  In5/1 -> diff30/1, diff29/1, diff28/1, diff27/1, diff22/2, diff17/2, diff11/2, diff4/2
  In6/1 -> diff33/1, diff32/1, diff31/1, diff27/2, diff23/2, diff18/2, diff12/2, diff5/2
  In7/1 -> diff19/2, diff35/1, diff34/1, diff31/2, diff28/2, diff24/2, diff13/2, diff6/2
  diff1/1 -> Logical Operator/1
  In3/1 -> diff2/2, diff21/1, diff20/1, diff19/1, diff18/1, diff17/1, diff16/1, diff9/2
  In4/1 -> diff26/1, diff25/1, diff24/1, diff23/1, diff22/1, diff16/2, diff10/2, diff3/2
  diff8/1 -> Logical Operator/8
  diff26/1 -> Logical Operator3/5
  diff36/1 -> Logical Operator7/1
  Logical Operator1/1 -> Logical Operator7/7
  diff10/1 -> Logical Operator1/2
  diff18/1 -> Logical Operator2/3
  diff17/1 -> Logical Operator2/2
  diff31/1 -> Logical Operator5/1
  Logical Operator5/1 -> Logical Operator7/3
  diff34/1 -> Logical Operator6/1
  diff16/1 -> Logical Operator2/1
  diff33/1 -> Logical Operator5/3
  diff22/1 -> Logical Operator3/1
  diff35/1 -> Logical Operator6/2
  diff27/1 -> Logical Operator4/1
  Logical Operator/1 -> Logical Operator7/8
  diff25/1 -> Logical Operator3/4
  diff3/1 -> Logical Operator/3
  diff2/1 -> Logical Operator/2
  diff7/1 -> Logical Operator/7
  diff5/1 -> Logical Operator/5
  diff4/1 -> Logical Operator/4
  diff30/1 -> Logical Operator4/4
  Logical Operator7/1 -> Out1/1
  Logical Operator3/1 -> Logical Operator7/5
  Logical Operator6/1 -> Logical Operator7/2
  diff14/1 -> Logical Operator1/6
  Logical Operator2/1 -> Logical Operator7/6
  diff15/1 -> Logical Operator1/7
  diff32/1 -> Logical Operator5/2
  diff21/1 -> Logical Operator2/6
  Logical Operator4/1 -> Logical Operator7/4
  diff19/1 -> Logical Operator2/4
  diff20/1 -> Logical Operator2/5
  diff28/1 -> Logical Operator4/2
  In8/1 -> diff29/2, diff36/1, diff34/2, diff32/2, diff25/2, diff20/2, diff14/2, diff7/2
  diff29/1 -> Logical Operator4/3
  diff6/1 -> Logical Operator/6
  diff9/1 -> Logical Operator1/1
  diff23/1 -> Logical Operator3/2
  diff13/1 -> Logical Operator1/5
  diff24/1 -> Logical Operator3/3
  diff11/1 -> Logical Operator1/3
  diff12/1 -> Logical Operator1/4
  In9/1 -> diff35/2, diff36/2, diff33/2, diff30/2, diff26/2, diff21/2, diff15/2, diff8/2

== system sudoku/columns/col_7 ==
  In1 : Inport
  In2 : Inport  Port=2
  In3 : Inport  Port=3
  In4 : Inport  Port=4
  In5 : Inport  Port=5
  In6 : Inport  Port=6
  In7 : Inport  Port=7
  In8 : Inport  Port=8
  In9 : Inport  Port=9
  Logical Operator : Logic  Inputs=8  AllPortsSameDT=off  OutDataTypeStr=boolean
  Logical Operator1 : Logic  Inputs=7  AllPortsSameDT=off  OutDataTypeStr=boolean
  Logical Operator2 : Logic  Inputs=6  AllPortsSameDT=off  OutDataTypeStr=boolean
  Logical Operator3 : Logic  Inputs=5  AllPortsSameDT=off  OutDataTypeStr=boolean
  Logical Operator4 : Logic  Inputs=4  AllPortsSameDT=off  OutDataTypeStr=boolean
  Logical Operator5 : Logic  Inputs=3  AllPortsSameDT=off  OutDataTypeStr=boolean
  Logical Operator6 : Logic  AllPortsSameDT=off  OutDataTypeStr=boolean
  Logical Operator7 : Logic  Inputs=8  AllPortsSameDT=off  OutDataTypeStr=boolean
  diff{1..36} (36 alike) : RelationalOperator  Operator=~=  OutDataTypeStr=boolean
  Out1 : Outport
  wires:
  In2/1 -> diff1/2, diff15/1, diff14/1, diff13/1, diff12/1, diff11/1, diff10/1, diff9/1
  In1/1 -> diff8/1, diff7/1, diff6/1, diff5/1, diff4/1, diff3/1, diff2/1, diff1/1
  In5/1 -> diff30/1, diff29/1, diff28/1, diff27/1, diff22/2, diff17/2, diff11/2, diff4/2
  In6/1 -> diff33/1, diff32/1, diff31/1, diff27/2, diff23/2, diff18/2, diff12/2, diff5/2
  In7/1 -> diff19/2, diff35/1, diff34/1, diff31/2, diff28/2, diff24/2, diff13/2, diff6/2
  diff1/1 -> Logical Operator/1
  In3/1 -> diff2/2, diff21/1, diff20/1, diff19/1, diff18/1, diff17/1, diff16/1, diff9/2
  In4/1 -> diff26/1, diff25/1, diff24/1, diff23/1, diff22/1, diff16/2, diff10/2, diff3/2
  diff8/1 -> Logical Operator/8
  diff26/1 -> Logical Operator3/5
  diff36/1 -> Logical Operator7/1
  Logical Operator1/1 -> Logical Operator7/7
  diff10/1 -> Logical Operator1/2
  diff18/1 -> Logical Operator2/3
  diff17/1 -> Logical Operator2/2
  diff31/1 -> Logical Operator5/1
  Logical Operator5/1 -> Logical Operator7/3
  diff34/1 -> Logical Operator6/1
  diff16/1 -> Logical Operator2/1
  diff33/1 -> Logical Operator5/3
  diff22/1 -> Logical Operator3/1
  diff35/1 -> Logical Operator6/2
  diff27/1 -> Logical Operator4/1
  Logical Operator/1 -> Logical Operator7/8
  diff25/1 -> Logical Operator3/4
  diff3/1 -> Logical Operator/3
  diff2/1 -> Logical Operator/2
  diff7/1 -> Logical Operator/7
  diff5/1 -> Logical Operator/5
  diff4/1 -> Logical Operator/4
  diff30/1 -> Logical Operator4/4
  Logical Operator7/1 -> Out1/1
  Logical Operator3/1 -> Logical Operator7/5
  Logical Operator6/1 -> Logical Operator7/2
  diff14/1 -> Logical Operator1/6
  Logical Operator2/1 -> Logical Operator7/6
  diff15/1 -> Logical Operator1/7
  diff32/1 -> Logical Operator5/2
  diff21/1 -> Logical Operator2/6
  Logical Operator4/1 -> Logical Operator7/4
  diff19/1 -> Logical Operator2/4
  diff20/1 -> Logical Operator2/5
  diff28/1 -> Logical Operator4/2
  In8/1 -> diff29/2, diff36/1, diff34/2, diff32/2, diff25/2, diff20/2, diff14/2, diff7/2
  diff29/1 -> Logical Operator4/3
  diff6/1 -> Logical Operator/6
  diff9/1 -> Logical Operator1/1
  diff23/1 -> Logical Operator3/2
  diff13/1 -> Logical Operator1/5
  diff24/1 -> Logical Operator3/3
  diff11/1 -> Logical Operator1/3
  diff12/1 -> Logical Operator1/4
  In9/1 -> diff35/2, diff36/2, diff33/2, diff30/2, diff26/2, diff21/2, diff15/2, diff8/2

== system sudoku/columns/col_8 ==
  In1 : Inport
  In2 : Inport  Port=2
  In3 : Inport  Port=3
  In4 : Inport  Port=4
  In5 : Inport  Port=5
  In6 : Inport  Port=6
  In7 : Inport  Port=7
  In8 : Inport  Port=8
  In9 : Inport  Port=9
  Logical Operator : Logic  Inputs=8  AllPortsSameDT=off  OutDataTypeStr=boolean
  Logical Operator1 : Logic  Inputs=7  AllPortsSameDT=off  OutDataTypeStr=boolean
  Logical Operator2 : Logic  Inputs=6  AllPortsSameDT=off  OutDataTypeStr=boolean
  Logical Operator3 : Logic  Inputs=5  AllPortsSameDT=off  OutDataTypeStr=boolean
  Logical Operator4 : Logic  Inputs=4  AllPortsSameDT=off  OutDataTypeStr=boolean
  Logical Operator5 : Logic  Inputs=3  AllPortsSameDT=off  OutDataTypeStr=boolean
  Logical Operator6 : Logic  AllPortsSameDT=off  OutDataTypeStr=boolean
  Logical Operator7 : Logic  Inputs=8  AllPortsSameDT=off  OutDataTypeStr=boolean
  diff{1..36} (36 alike) : RelationalOperator  Operator=~=  OutDataTypeStr=boolean
  Out1 : Outport
  wires:
  In2/1 -> diff1/2, diff15/1, diff14/1, diff13/1, diff12/1, diff11/1, diff10/1, diff9/1
  In1/1 -> diff8/1, diff7/1, diff6/1, diff5/1, diff4/1, diff3/1, diff2/1, diff1/1
  In5/1 -> diff30/1, diff29/1, diff28/1, diff27/1, diff22/2, diff17/2, diff11/2, diff4/2
  In6/1 -> diff33/1, diff32/1, diff31/1, diff27/2, diff23/2, diff18/2, diff12/2, diff5/2
  In7/1 -> diff19/2, diff35/1, diff34/1, diff31/2, diff28/2, diff24/2, diff13/2, diff6/2
  diff1/1 -> Logical Operator/1
  In3/1 -> diff2/2, diff21/1, diff20/1, diff19/1, diff18/1, diff17/1, diff16/1, diff9/2
  In4/1 -> diff26/1, diff25/1, diff24/1, diff23/1, diff22/1, diff16/2, diff10/2, diff3/2
  diff8/1 -> Logical Operator/8
  diff26/1 -> Logical Operator3/5
  diff36/1 -> Logical Operator7/1
  Logical Operator1/1 -> Logical Operator7/7
  diff10/1 -> Logical Operator1/2
  diff18/1 -> Logical Operator2/3
  diff17/1 -> Logical Operator2/2
  diff31/1 -> Logical Operator5/1
  Logical Operator5/1 -> Logical Operator7/3
  diff34/1 -> Logical Operator6/1
  diff16/1 -> Logical Operator2/1
  diff33/1 -> Logical Operator5/3
  diff22/1 -> Logical Operator3/1
  diff35/1 -> Logical Operator6/2
  diff27/1 -> Logical Operator4/1
  Logical Operator/1 -> Logical Operator7/8
  diff25/1 -> Logical Operator3/4
  diff3/1 -> Logical Operator/3
  diff2/1 -> Logical Operator/2
  diff7/1 -> Logical Operator/7
  diff5/1 -> Logical Operator/5
  diff4/1 -> Logical Operator/4
  diff30/1 -> Logical Operator4/4
  Logical Operator7/1 -> Out1/1
  Logical Operator3/1 -> Logical Operator7/5
  Logical Operator6/1 -> Logical Operator7/2
  diff14/1 -> Logical Operator1/6
  Logical Operator2/1 -> Logical Operator7/6
  diff15/1 -> Logical Operator1/7
  diff32/1 -> Logical Operator5/2
  diff21/1 -> Logical Operator2/6
  Logical Operator4/1 -> Logical Operator7/4
  diff19/1 -> Logical Operator2/4
  diff20/1 -> Logical Operator2/5
  diff28/1 -> Logical Operator4/2
  In8/1 -> diff29/2, diff36/1, diff34/2, diff32/2, diff25/2, diff20/2, diff14/2, diff7/2
  diff29/1 -> Logical Operator4/3
  diff6/1 -> Logical Operator/6
  diff9/1 -> Logical Operator1/1
  diff23/1 -> Logical Operator3/2
  diff13/1 -> Logical Operator1/5
  diff24/1 -> Logical Operator3/3
  diff11/1 -> Logical Operator1/3
  diff12/1 -> Logical Operator1/4
  In9/1 -> diff35/2, diff36/2, diff33/2, diff30/2, diff26/2, diff21/2, diff15/2, diff8/2

== system sudoku/columns/col_9 ==
  In1 : Inport
  In2 : Inport  Port=2
  In3 : Inport  Port=3
  In4 : Inport  Port=4
  In5 : Inport  Port=5
  In6 : Inport  Port=6
  In7 : Inport  Port=7
  In8 : Inport  Port=8
  In9 : Inport  Port=9
  Logical Operator : Logic  Inputs=8  AllPortsSameDT=off  OutDataTypeStr=boolean
  Logical Operator1 : Logic  Inputs=7  AllPortsSameDT=off  OutDataTypeStr=boolean
  Logical Operator2 : Logic  Inputs=6  AllPortsSameDT=off  OutDataTypeStr=boolean
  Logical Operator3 : Logic  Inputs=5  AllPortsSameDT=off  OutDataTypeStr=boolean
  Logical Operator4 : Logic  Inputs=4  AllPortsSameDT=off  OutDataTypeStr=boolean
  Logical Operator5 : Logic  Inputs=3  AllPortsSameDT=off  OutDataTypeStr=boolean
  Logical Operator6 : Logic  AllPortsSameDT=off  OutDataTypeStr=boolean
  Logical Operator7 : Logic  Inputs=8  AllPortsSameDT=off  OutDataTypeStr=boolean
  diff{1..36} (36 alike) : RelationalOperator  Operator=~=  OutDataTypeStr=boolean
  Out1 : Outport
  wires:
  In2/1 -> diff1/2, diff15/1, diff14/1, diff13/1, diff12/1, diff11/1, diff10/1, diff9/1
  In1/1 -> diff8/1, diff7/1, diff6/1, diff5/1, diff4/1, diff3/1, diff2/1, diff1/1
  In5/1 -> diff30/1, diff29/1, diff28/1, diff27/1, diff22/2, diff17/2, diff11/2, diff4/2
  In6/1 -> diff33/1, diff32/1, diff31/1, diff27/2, diff23/2, diff18/2, diff12/2, diff5/2
  In7/1 -> diff19/2, diff35/1, diff34/1, diff31/2, diff28/2, diff24/2, diff13/2, diff6/2
  diff1/1 -> Logical Operator/1
  In3/1 -> diff2/2, diff21/1, diff20/1, diff19/1, diff18/1, diff17/1, diff16/1, diff9/2
  In4/1 -> diff26/1, diff25/1, diff24/1, diff23/1, diff22/1, diff16/2, diff10/2, diff3/2
  diff8/1 -> Logical Operator/8
  diff26/1 -> Logical Operator3/5
  diff36/1 -> Logical Operator7/1
  Logical Operator1/1 -> Logical Operator7/7
  diff10/1 -> Logical Operator1/2
  diff18/1 -> Logical Operator2/3
  diff17/1 -> Logical Operator2/2
  diff31/1 -> Logical Operator5/1
  Logical Operator5/1 -> Logical Operator7/3
  diff34/1 -> Logical Operator6/1
  diff16/1 -> Logical Operator2/1
  diff33/1 -> Logical Operator5/3
  diff22/1 -> Logical Operator3/1
  diff35/1 -> Logical Operator6/2
  diff27/1 -> Logical Operator4/1
  Logical Operator/1 -> Logical Operator7/8
  diff25/1 -> Logical Operator3/4
  diff3/1 -> Logical Operator/3
  diff2/1 -> Logical Operator/2
  diff7/1 -> Logical Operator/7
  diff5/1 -> Logical Operator/5
  diff4/1 -> Logical Operator/4
  diff30/1 -> Logical Operator4/4
  Logical Operator7/1 -> Out1/1
  Logical Operator3/1 -> Logical Operator7/5
  Logical Operator6/1 -> Logical Operator7/2
  diff14/1 -> Logical Operator1/6
  Logical Operator2/1 -> Logical Operator7/6
  diff15/1 -> Logical Operator1/7
  diff32/1 -> Logical Operator5/2
  diff21/1 -> Logical Operator2/6
  Logical Operator4/1 -> Logical Operator7/4
  diff19/1 -> Logical Operator2/4
  diff20/1 -> Logical Operator2/5
  diff28/1 -> Logical Operator4/2
  In8/1 -> diff29/2, diff36/1, diff34/2, diff32/2, diff25/2, diff20/2, diff14/2, diff7/2
  diff29/1 -> Logical Operator4/3
  diff6/1 -> Logical Operator/6
  diff9/1 -> Logical Operator1/1
  diff23/1 -> Logical Operator3/2
  diff13/1 -> Logical Operator1/5
  diff24/1 -> Logical Operator3/3
  diff11/1 -> Logical Operator1/3
  diff12/1 -> Logical Operator1/4
  In9/1 -> diff35/2, diff36/2, diff33/2, diff30/2, diff26/2, diff21/2, diff15/2, diff8/2
